simulink model "Lorenz"  (R2018b)
settings: Solver=ode45  StartTime=0.0  StopTime=50  RelTol=1e-3
settings Model: Creator=12732  LastModifiedBy=12732
settings DataIOCC: SaveFormat=Array

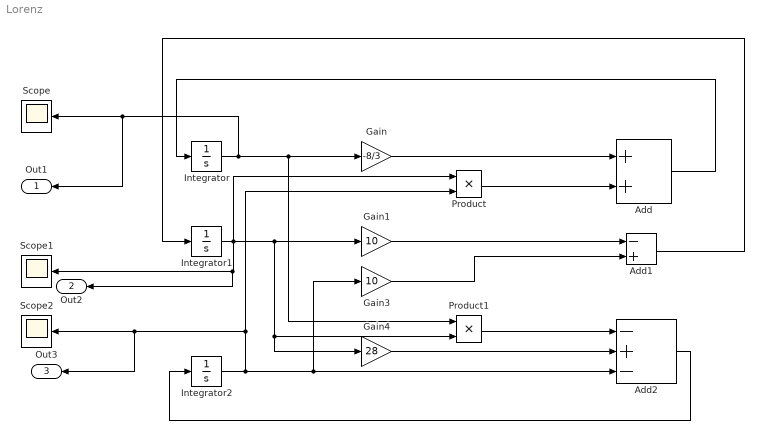
== system Lorenz ==
  Add : Sum
  Add1 : Sum  Inputs=-+
  Add2 : Sum  Inputs=-+-
  Gain : Gain  Gain=-8/3
  Gain1 : Gain  Gain=10
  Gain3 : Gain  Gain=10
  Gain4 : Gain  Gain=28
  Integrator : Integrator
  Integrator1 : Integrator
  Integrator2 : Integrator  InitialCondition=1e-10
  Product : Product
  Product1 : Product
  Scope : Scope
  Scope1 : Scope
  Scope2 : Scope
  Out1 : Outport
  Out2 : Outport  Port=2
  Out3 : Outport  Port=3
  wires:
  Integrator/1 -> Out1/1, Scope/1, Product1/1, Gain/1
  Gain/1 -> Add/1
  Integrator1/1 -> Product/1, Out2/1, Scope1/1, Gain4/1, Product1/2, Gain1/1
  Integrator2/1 -> Product/2, Out3/1, Scope2/1, Gain3/1, Add2/3
  Add/1 -> Integrator/1
  Product/1 -> Add/2
  Gain1/1 -> Add1/1
  Gain3/1 -> Add1/2
  Add1/1 -> Integrator1/1
  Product1/1 -> Add2/1
  Gain4/1 -> Add2/2
  Add2/1 -> Integrator2/1
